simulink model "testPSP"  (R2018a)
settings: Solver=VariableStepAuto  StartTime=0.0  StopTime=10.0  RelTol=1e-3
undefined symbols (not defined in the file or in its folder): LPwraparm
settings Model: Creator=Meng Chaoheng  LastModifiedBy=Meng Chaoheng

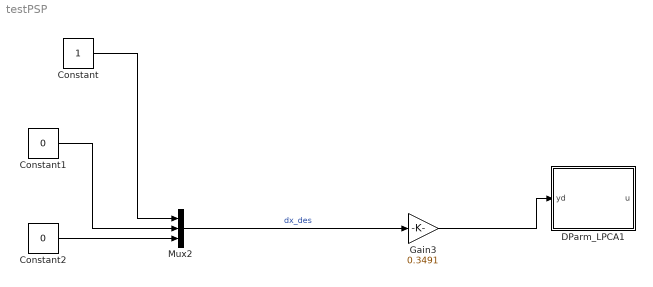
== system testPSP ==
  Constant : Constant
  Constant1 : Constant  Value=0
  Constant2 : Constant  Value=0
  DParm_LPCA1 : Subsystem
  Gain3 : Gain  Gain=0.3491
  Mux2 : Mux  Inputs=3
  wires:
  Constant2/1 -> Mux2/3
  Constant/1 -> Mux2/1
  Constant1/1 -> Mux2/2
  Gain3/1 -> DParm_LPCA1/1(yd)
  Mux2/1 -> Gain3/1  "dx_des"

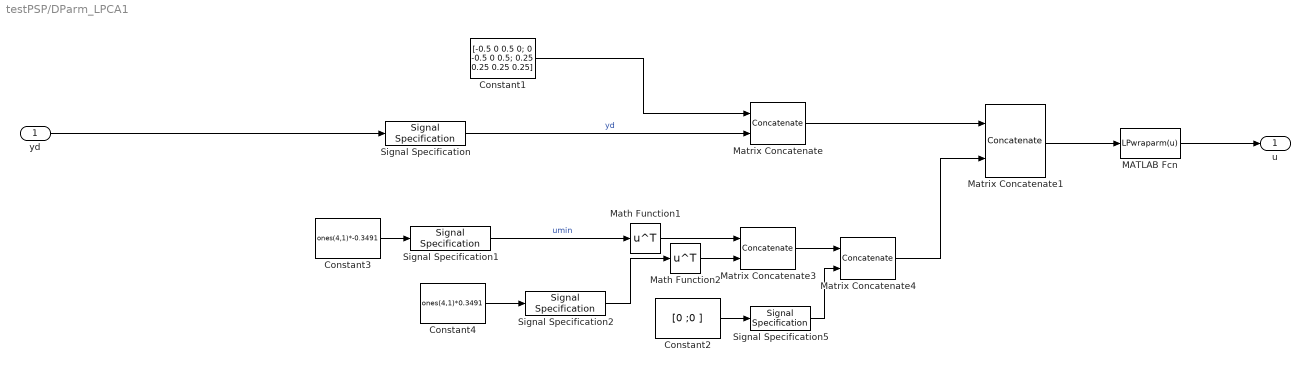
== system testPSP/DParm_LPCA1 ==
  yd : Inport
  Constant1 : Constant  Value=|
      | [-0.5     0       0.5     0;
      |                      0      -0.5     0       0.5;
      |                      0.25    0.25    0.25    0.25]
  Constant2 : Constant  Value=[0 ;0 ]
  Constant3 : Constant  Value=ones(4,1)*-0.3491
  Constant4 : Constant  Value=ones(4,1)*0.3491
  MATLAB Fcn : MATLABFcn  MATLABFcn=LPwraparm(u)
  Math Function1 : Math  Operator=transpose  SaturateOnIntegerOverflow=on
  Math Function2 : Math  Operator=transpose  SaturateOnIntegerOverflow=on
  Matrix Concatenate : Concatenate  Mode=Multidimensional array  ConcatenateDimension=2
  Matrix Concatenate1 : Concatenate  Mode=Multidimensional array
  Matrix Concatenate3 : Concatenate  Mode=Multidimensional array
  Matrix Concatenate4 : Concatenate  Mode=Multidimensional array  ConcatenateDimension=2
  Signal Specification : SignalSpecification  Dimensions=[3 1]
  Signal Specification1 : SignalSpecification  Dimensions=[4 1]
  Signal Specification2 : SignalSpecification  Dimensions=[4 1]
  Signal Specification5 : SignalSpecification  Dimensions=[2 1]
  u : Outport
  wires:
  Math Function1/1 -> Matrix Concatenate3/1
  Matrix Concatenate1/1 -> MATLAB Fcn/1
  Signal Specification2/1 -> Math Function2/1
  Signal Specification5/1 -> Matrix Concatenate4/2
  Matrix Concatenate3/1 -> Matrix Concatenate4/1
  Matrix Concatenate/1 -> Matrix Concatenate1/1
  Signal Specification1/1 -> Math Function1/1  "umin"
  Matrix Concatenate4/1 -> Matrix Concatenate1/2
  yd/1 -> Signal Specification/1
  MATLAB Fcn/1 -> u/1
  Constant1/1 -> Matrix Concatenate/1
  Constant2/1 -> Signal Specification5/1
  Signal Specification/1 -> Matrix Concatenate/2  "yd"
  Constant4/1 -> Signal Specification2/1
  Math Function2/1 -> Matrix Concatenate3/2
  Constant3/1 -> Signal Specification1/1
